simulink model "draft"  (R2022a)
settings: Solver=FixedStepAuto  StartTime=0.0  StopTime=10.0  FixedStep=1/60  RelTol=1e-3
model workspace (MAT data in the model file):
  Sig = Simulink.Signal
  Sig.DataType = 'auto'
  Sig.Dimensions = -1
  Sig.DimensionsMode = 'auto'
  Sig.Complexity = 'auto'
  Sig.SampleTime = -1
  Sig.SamplingMode = 'auto'
  control = Simulink.Parameter
  control.Value = 1
  control.DataType = 'int8'
  control.Complexity = 'real'
  control.Dimensions = [1 1]
  gscore_array = Simulink.Parameter
  gscore_array.Value = [17 110 46 69 87 122 39 120 84 96 127 126 70 103 21 90 10 59 100 91 32 54 112 72 40 107 52 16 61 89 102 14 44 80 29 119 121 81 30 118 62 76 50 12 94 88 43 71 109 27 47 22 115 64 77 99 66 31 58 2 101 51 123 57 25 73 41 83 37 26 35 67 98 6 75 36 34 78 125 45 19 56 5 92 9 68 95 42 4 85 60 74 82 105 124 53 20 97 13 128 3 86 33 79 48 55 23 38 49 63 11 104 24 15 7 18 117 28 114 106 65 108 93 8 1 116 113 111]
  gscore_array.DataType = 'int32'
  gscore_array.Complexity = 'real'
  gscore_array.Dimensions = [1 128]
  id_array = Simulink.Parameter
  id_array.Value = [122 98 15 34 91 1 90 8 53 118 126 37 120 59 76 61 100 114 71 77 46 30 45 13 85 112 75 106 80 23 47 102 42 128 52 12 66 79 33 4 17 10 2 32 63 97 21 82 92 110 127 51 119 56 103 16 26 64 72 5 41 9 116 105 19 87 6 81 74 107 28 70 93 40 108 18 57 84 14 35 101 109 60 38 22 49 86 94 48 54 29 78 69 58 115 123 83 39 88 24 27 124 96 113 7 55 50 11 125 20 67 36 73 104 3 65 121 111 44 95 117 31 25 62 43 68 89 99]
  id_array.DataType = 'int8'
  id_array.Complexity = 'real'
  id_array.Dimensions = [1 128]
  pscore_array = Simulink.Parameter
  pscore_array.Value = [46 24 47 116 19 62 17 9 48 113 58 100 108 34 36 90 54 96 1 86 91 59 25 107 26 84 101 104 121 126 13 65 109 51 16 110 50 60 40 57 95 102 6 99 80 5 42 111 82 64 81 41 23 11 18 122 112 72 119 22 75 103 127 105 49 125 27 124 10 120 63 56 61 87 35 106 30 66 69 128 28 21 12 33 76 2 118 97 68 44 89 85 115 78 92 88 98 83 14 31 7 20 38 77 45 55 52 8 117 70 73 32 29 67 74 37 3 94 123 79 93 43 71 4 53 114 15 39]
  pscore_array.DataType = 'int32'
  pscore_array.Complexity = 'real'
  pscore_array.Dimensions = [1 128]
  size_array = Simulink.Parameter
  size_array.Value = [26 78 48 106 88 64 41 23 81 6 15 66 8 103 121 14 83 114 102 40 110 45 118 5 90 10 67 123 96 57 82 126 47 77 27 7 127 72 91 94 111 84 52 53 117 11 4 124 74 2 119 112 9 99 37 69 68 120 16 3 107 50 21 1 55 98 62 101 97 100 33 122 125 60 116 44 38 79 128 29 87 86 24 42 71 73 65 93 17 12 59 25 70 95 54 108 18 89 115 51 58 31 80 104 13 49 34 85 43 35 113 63 36 105 32 46 19 76 92 20 28 30 61 75 109 22 56 39]
  size_array.DataType = 'int8'
  size_array.Complexity = 'real'
  size_array.Dimensions = [1 128]
  tag_array = ["happy" "hour" "sorry" "maker" "hi"]
  x_array = Simulink.Parameter
  x_array.Value = [70 27 78 58 7 16 43 13 93 9 22 42 106 79 124 59 85 91 35 45 2 103 6 89 105 49 92 19 83 1 117 20 122 73 11 5 77 56 81 123 67 97 48 65 30 3 10 114 108 64 109 84 96 18 94 33 74 80 55 76 127 44 47 98 120 26 61 100 90 119 51 39 118 104 113 8 54 17 60 41 88 128 25 15 40 111 63 21 38 52 12 68 28 29 31 62 116 86 95 32 99 36 87 24 75 121 101 14 34 23 69 57 46 50 102 115 72 125 66 107 82 71 112 4 110 53 37 126]
  x_array.DataType = 'int16'
  x_array.Complexity = 'real'
  x_array.Dimensions = [1 128]
  y_array = Simulink.Parameter
  y_array.Value = [100 36 126 20 33 91 7 83 1 116 51 85 24 90 41 127 88 39 19 34 64 55 60 5 107 81 25 40 114 26 44 77 12 29 8 10 15 72 13 37 2 18 52 87 89 4 58 54 46 62 105 31 93 108 104 96 53 11 86 63 70 27 102 110 73 79 113 30 32 50 71 123 125 117 69 48 115 118 92 97 21 74 112 38 106 78 119 101 59 61 14 6 68 122 42 67 49 99 109 47 94 103 57 9 16 75 120 22 82 80 128 3 95 66 45 124 65 28 121 17 98 111 35 84 56 23 76 43]
  y_array.DataType = 'int16'
  y_array.Complexity = 'real'
  y_array.Dimensions = [1 128]
undefined symbols (not defined in the file): player_id, timestamp, x, y
libraries: ros2lib x15
settings Model: PacingRate=0.100000  Creator=ifate  LastModifiedBy=ifate
settings DataIOCC: InspectSignalLogs=on
settings OptimizationCC: EnhancedBackFolding=on  PassReuseOutputArgsAs=Individual arguments  ZeroExternalMemoryAtStartup=off  ZeroInternalMemoryAtStartup=off  MaxStackSize=64  OptimizeBlockOrder=speed  DifferentSizesBufferReuse=on  OptimizationCustomize=off  EfficientTunableParamExpr=on
settings DebuggingCC: ParameterTunabilityLossMsg=error
settings HardwareCC: UseEmbeddedCoderFeatures=off
settings SFSimCC: MATLABDynamicMemAlloc=off
settings RTWCC: SystemTargetFile=ert.tlc  HardwareBoard=Robot Operating System 2 (ROS 2)  TLCOptions="-aInlineSetEventsForThisBaseRateFcn=TLC_FALSE -aSuppressMultiTaskScheduler=TLC_FALSE  -aRateBasedStepFcn=0"  TemplateMakefile=ert_default_tmf  Toolchain=Colcon Tools  TargetLang=C++
settings CodeAppCC: ForceParamTrailComments=on  IgnoreCustomStorageClasses=off  OperatorAnnotations=on  SimulinkDataObjDesc=on  SFDataObjDesc=on  InsertBlockDesc=on
settings ERTTargetCC: CodeInterfacePackaging=C++ class  SupportNonInlinedSFcns=on  RootIOFormat=Structure reference

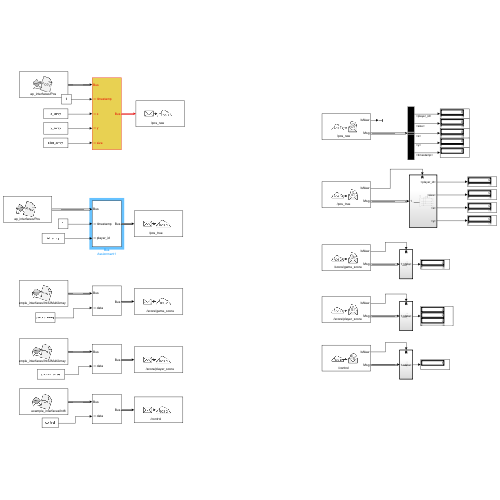
[thumbnail: Simulink's stored preview of the top-level diagram]
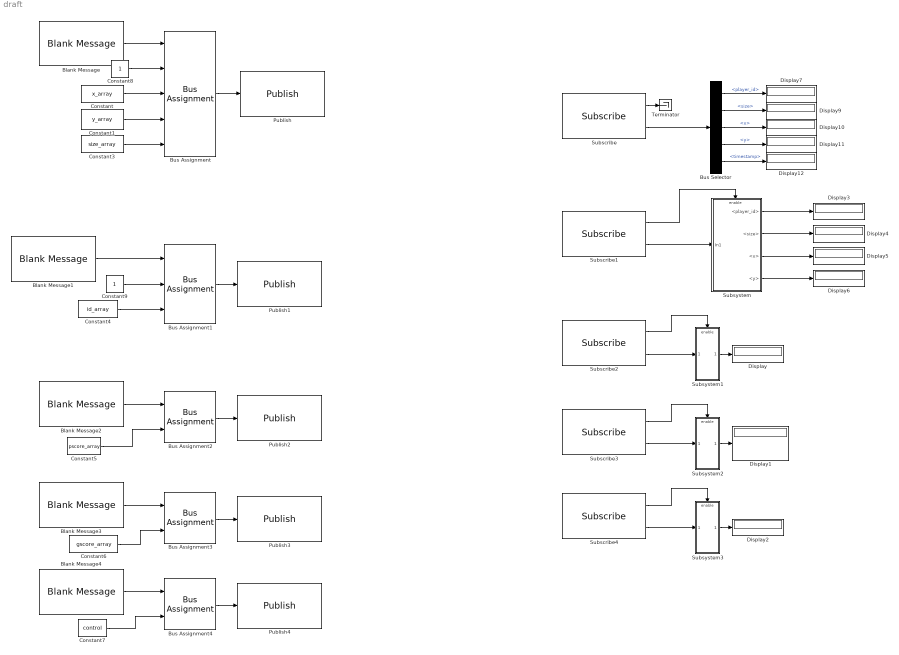
== system draft ==
  Blank Message : ros2lib/Blank Message  messageClass=Message  entityType=ap_interfaces/Pos  messageType=ap_interfaces/Pos  SampleTime=1/60
      settings: SourceProductBaseCode=RR
  Blank Message1 : ros2lib/Blank Message  messageClass=Message  entityType=ap_interfaces/Pos  messageType=ap_interfaces/Pos  SampleTime=1/60
      settings: SourceProductBaseCode=RR
  Blank Message2 : ros2lib/Blank Message  messageClass=Message  entityType=example_interfaces/Int32MultiArray  messageType=example_interfaces/Int32MultiArray  SampleTime=1/60
      settings: SourceProductBaseCode=RR
  Blank Message3 : ros2lib/Blank Message  messageClass=Message  entityType=example_interfaces/Int32MultiArray  messageType=example_interfaces/Int32MultiArray  SampleTime=1/60
      settings: SourceProductBaseCode=RR
  Blank Message4 : ros2lib/Blank Message  messageClass=Message  entityType=example_interfaces/Int8  messageType=example_interfaces/Int8  SampleTime=1/60
      settings: SourceProductBaseCode=RR
  Bus Assignment : BusAssignment  AssignedSignals=timestamp,x,y,size
  Bus Assignment1 : BusAssignment  AssignedSignals=timestamp,player_id
  Bus Assignment2 : BusAssignment  AssignedSignals=data
  Bus Assignment3 : BusAssignment  AssignedSignals=data
  Bus Assignment4 : BusAssignment  AssignedSignals=data
  Bus Selector : BusSelector  OutputSignals=player_id,size,x,y,timestamp
  Constant : Constant  Value=x_array
  Constant1 : Constant  Value=y_array
  Constant3 : Constant  Value=size_array
  Constant4 : Constant  Value=id_array
  Constant5 : Constant  Value=pscore_array
  Constant6 : Constant  Value=gscore_array
  Constant7 : Constant  Value=control
  Constant8 : Constant
  Constant9 : Constant
  Display{,1..7,9..12} (12 alike) : Display
  Publish : ros2lib/Publish  topicSource=Specify your own  topic=/pos_raw  messageType=ap_interfaces/Pos  QOSHistory=Keep last  QOSDepth=1  QOSReliability=Reliable  QOSDurability=Volatile
      settings: SourceProductBaseCode=RR
  Publish1 : ros2lib/Publish  topicSource=Specify your own  topic=/pos_true  messageType=ap_interfaces/Pos  QOSHistory=Keep last  QOSDepth=1  QOSReliability=Reliable  QOSDurability=Volatile
      settings: SourceProductBaseCode=RR
  Publish2 : ros2lib/Publish  topicSource=Specify your own  topic=/score/game_score  messageType=example_interfaces/Int32MultiArray  QOSHistory=Keep last  QOSDepth=1  QOSReliability=Reliable  QOSDurability=Volatile
      settings: SourceProductBaseCode=RR
  Publish3 : ros2lib/Publish  topicSource=Specify your own  topic=/score/player_score  messageType=example_interfaces/Int32MultiArray  QOSHistory=Keep last  QOSDepth=1  QOSReliability=Reliable  QOSDurability=Volatile
      settings: SourceProductBaseCode=RR
  Publish4 : ros2lib/Publish  topicSource=Specify your own  topic=/control  messageType=example_interfaces/Int8  QOSHistory=Keep last  QOSDepth=1  QOSReliability=Reliable  QOSDurability=Volatile
      settings: SourceProductBaseCode=RR
  Subscribe : ros2lib/Subscribe  topicSource=Specify your own  topic=/pos_raw  messageType=ap_interfaces/Pos  sampleTime=inf  QOSHistory=Keep last  QOSDepth=1  QOSReliability=Reliable  QOSDurability=Volatile
      settings: SourceProductBaseCode=RR
  Subscribe1 : ros2lib/Subscribe  topicSource=Specify your own  topic=/pos_true  messageType=ap_interfaces/Pos  sampleTime=1/60  QOSHistory=Keep last  QOSDepth=1  QOSReliability=Reliable  QOSDurability=Volatile
      settings: SourceProductBaseCode=RR
  Subscribe2 : ros2lib/Subscribe  topicSource=Specify your own  topic=/score/game_score  messageType=example_interfaces/Int32MultiArray  sampleTime=1/60  QOSHistory=Keep last  QOSDepth=1  QOSReliability=Reliable  QOSDurability=Volatile
      settings: SourceProductBaseCode=RR
  Subscribe3 : ros2lib/Subscribe  topicSource=Specify your own  topic=/score/player_score  messageType=example_interfaces/Int32MultiArray  sampleTime=1/60  QOSHistory=Keep last  QOSDepth=1  QOSReliability=Reliable  QOSDurability=Volatile
      settings: SourceProductBaseCode=RR
  Subscribe4 : ros2lib/Subscribe  topicSource=Specify your own  topic=/control  messageType=example_interfaces/Int8  sampleTime=1/60  QOSHistory=Keep last  QOSDepth=1  QOSReliability=Reliable  QOSDurability=Volatile
      settings: SourceProductBaseCode=RR
  Subsystem : Subsystem
  Subsystem1 : Subsystem
  Subsystem2 : Subsystem
  Subsystem3 : Subsystem
  Terminator : Terminator
  wires:
  Blank Message/1 -> Bus Assignment/1
  Bus Assignment/1 -> Publish/1
  Blank Message1/1 -> Bus Assignment1/1
  Bus Assignment1/1 -> Publish1/1
  Blank Message2/1 -> Bus Assignment2/1
  Bus Assignment2/1 -> Publish2/1
  Bus Assignment3/1 -> Publish3/1
  Blank Message3/1 -> Bus Assignment3/1
  Subscribe/2 -> Bus Selector/1
  Blank Message4/1 -> Bus Assignment4/1
  Bus Assignment4/1 -> Publish4/1
  Constant8/1 -> Bus Assignment/2
  Constant9/1 -> Bus Assignment1/2
  Subscribe1/2 -> Subsystem/1(In1)
  Subsystem/1(<player_id>) -> Display3/1
  Subsystem/2(<size>) -> Display4/1
  Subsystem/3(<x>) -> Display5/1
  Subsystem/4(<y>) -> Display6/1
  Subscribe1/1 -> Subsystem/Enable
  Subscribe2/2 -> Subsystem1/1(In1)
  Subsystem1/1(<data>) -> Display/1
  Subscribe2/1 -> Subsystem1/Enable
  Subscribe3/2 -> Subsystem2/1(In1)
  Subsystem2/1(<data>) -> Display1/1
  Subscribe3/1 -> Subsystem2/Enable
  Subscribe4/2 -> Subsystem3/1(In1)
  Subsystem3/1(<data>) -> Display2/1
  Subscribe4/1 -> Subsystem3/Enable
  Subscribe/1 -> Terminator/1
  Constant/1 -> Bus Assignment/3
  Constant1/1 -> Bus Assignment/4
  Constant3/1 -> Bus Assignment/5
  Constant4/1 -> Bus Assignment1/3
  Constant5/1 -> Bus Assignment2/2
  Constant6/1 -> Bus Assignment3/2
  Constant7/1 -> Bus Assignment4/2
  Bus Selector/1 -> Display7/1  "<player_id>"
  Bus Selector/2 -> Display9/1  "<size>"
  Bus Selector/3 -> Display10/1  "<x>"
  Bus Selector/4 -> Display11/1  "<y>"
  Bus Selector/5 -> Display12/1  "<timestamp>"

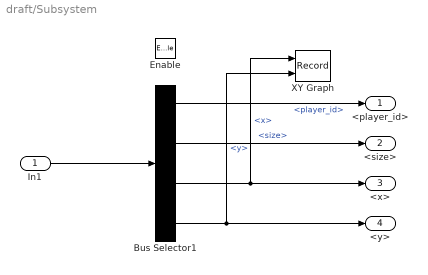
== system draft/Subsystem ==
  In1 : Inport
  Enable : EnablePort
  Bus Selector1 : BusSelector  OutputSignals=player_id,size,x,y
  XY Graph : Record  FileSettingsInternal="{\"entries\":[{\"content\":{\"excelSettings\":{\"content\":{},\"type\":\"Streamout.ExcelSettings\"}},\"type\":\"Streamout.FileSettingStorage\",\"uuid\":\"ebdd8d9c-e8d9-40ac-b7ed-b3f8572c778b\"}],\"packageUris\":[\"http://schema.mathworks.com/mf0/streamout_blocks/R2020a\"],\"version\":\"1.0\"}"  Layout=[1 1]  SignalsInternal="{\"entries\":[{\"content\":{\"signals\":[{\"content\":{\"blockPath\":[\"draft/Subsystem/XY Graph\"],\"channel\":[],\"dimensions\":[128],\"domain\":\"draft/Subsystem/XY Graph\",\"hasChildren\":true,\"lineColor\":\"#22b573\",\"plots\":[],\"port\":1,\"sid\":[\"\"],\"signalID\":623,\"signalName\":\"<x>\"},\"type\":\"RecordBlkView.Signal\",\"uuid\":\"cde3b60e-2d79-4b0b-9062-66c1d8791405\"},{\"content\":{\"blockPath\":[\"draft/Subsystem/XY Graph\"],\"channel\":[1],\"dimensions\":[128],\"domain\":\"draft/Subsystem/XY Graph\",\"lineColor\":\"#0072bd\",\"parentID\":623,\"plots\":[],\"port\":1,\"sid\":[\"\"],\"signalID\":624,\"signalName\":\"<x>\"},\"type\":\"RecordBlkView.Signal\",\"uuid\":\"5aff8c8a-40f7-49dc-b977-27caabb62910\"},{\"content\":{\"blockPath\":[\"draft/Subsystem/XY Graph\"],\"channel\":[],\"dimensions\":[128],\"domain\":\"draft/Subsystem/XY Graph\",\"hasChildren\":true,\"lineColor\":\"#d95319\",\"plots\":[],\"port\":2,\"sid\":[\"\"],\"signalID\":628,\"signalName\":\"<y>\"},\"type\":\"RecordBlkView.Signal\",\"uuid\":\"91b67a6a-6798-4c30-9fcf-07dd5c9425c3\"},{\"content\":{\"blockPath\":[\"draft/Subsystem/XY Graph\"],\"channel\":[1],\"dimensions\":[128],\"domain\":\"draft/Subsystem/XY Graph\",\"lineColor\":\"#edb120\",\"parentID\":628,\"plots\":[],\"port\":2,\"sid\":[\"\"],\"signalID\":629,\"signalName\":\"<y>\"},\"type\":\"RecordBlkView.Signal\",\"uuid\":\"793540aa-1bb9-4611-8d87-558853c061e1\"}]},\"type\":\"RecordBlkView.InputSignals\",\"uuid\":\"dd062b24-844b-4a39-a3a4-2c3045f44376\"}],\"packageUris\":[\"http://schema.mathworks.com/mf0/streamout_blocks/R2020a\"],\"version\":\"1.0\"}"  VisualizationBindings="{\"xyplotplugin\":{\"info\":[{\"series\":[],\"subplotID\":1}]}}"  CompatibilityTag=XY
  <player_id> : Outport
  <size> : Outport  Port=2
  <x> : Outport  Port=3
  <y> : Outport  Port=4
  wires:
  Bus Selector1/4 -> <y>/1, XY Graph/2  "<y>"
  Bus Selector1/3 -> <x>/1, XY Graph/1  "<x>"
  Bus Selector1/2 -> <size>/1  "<size>"
  In1/1 -> Bus Selector1/1
  Bus Selector1/1 -> <player_id>/1  "<player_id>"

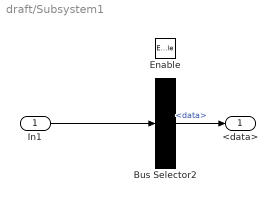
== system draft/Subsystem1 ==
  In1 : Inport
  Enable : EnablePort
  Bus Selector2 : BusSelector  OutputSignals=data
  <data> : Outport
  wires:
  In1/1 -> Bus Selector2/1
  Bus Selector2/1 -> <data>/1  "<data>"

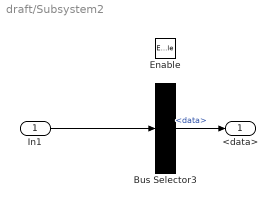
== system draft/Subsystem2 ==
  In1 : Inport
  Enable : EnablePort
  Bus Selector3 : BusSelector  OutputSignals=data
  <data> : Outport
  wires:
  Bus Selector3/1 -> <data>/1  "<data>"
  In1/1 -> Bus Selector3/1

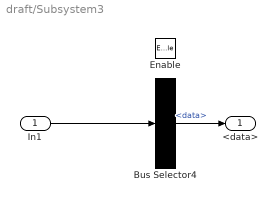
== system draft/Subsystem3 ==
  In1 : Inport
  Enable : EnablePort
  Bus Selector4 : BusSelector  OutputSignals=data
  <data> : Outport
  wires:
  Bus Selector4/1 -> <data>/1  "<data>"
  In1/1 -> Bus Selector4/1
